simulink model "A1_acc_R2017b"  (R2017b)
settings: Solver=ode45  StartTime=0.0  StopTime=80.0  MaxStep=0.001  RelTol=1e-3
values from neighbouring files (symbols this model uses):
  a = data(2)    [A1_10.m]    (also in problem6.m = 270)
  b = data(3)    [A1_10.m]    (also in problem6.m = 11000)
  Ki = 0.0    (= 0)    [A1_10.m]
  Kp = 0.0    (= 0)    [A1_10.m]
  m = data(1)    [A1_10.m]    (also in problem6.m = 1740)
undefined symbols (not defined in the file or in its folder): Kd
settings Model: Creator=jofr  LastModifiedBy=jofr
settings DataIOCC: LimitDataPoints=on  SaveFormat=Array  SignalLoggingSaveFormat=ModelDataLogs
settings OptimizationCC: BlockReduction=off  BooleanDataType=off  LifeSpan=inf
settings DebuggingCC: SaveWithParameterizedLinksMsg=none  UnderspecifiedInitializationDetection=Classic  MergeDetectMultiDrivingBlocksExec=none  SignalResolutionControl=TryResolveAllWithWarning  MultiTaskDSMMsg=warning  MultiTaskCondExecSysMsg=none  SFUnexpectedBacktrackingDiag=warning  SFNoUnconditionalDefaultTransitionDiag=warning  SFExecutionAtInitializationDiag=none
settings HardwareCC: ProdBitPerPointer=32  ProdBitPerSizeT=32  ProdBitPerPtrDiffT=32  ProdLargestAtomicFloat=None  ProdIntDivRoundTo=Undefined  ProdEndianess=Unspecified  ProdWordSize=32  ProdHWDeviceType=32-bit Generic  TargetUnknown=on
settings ModelReferenceCC: PropagateSignalLabelsOutOfModel=off
settings CodeAppCC: StateflowObjectComments=on
settings GRTTargetCC: TargetLangStandard=C89/C90 (ANSI)
settings ConfigComp: CovMetricSettings=dw  CovSaveCumulativeToWorkspaceVar=on  CovSaveSingleToWorkspaceVar=on  CovExternalEMLEnable=off

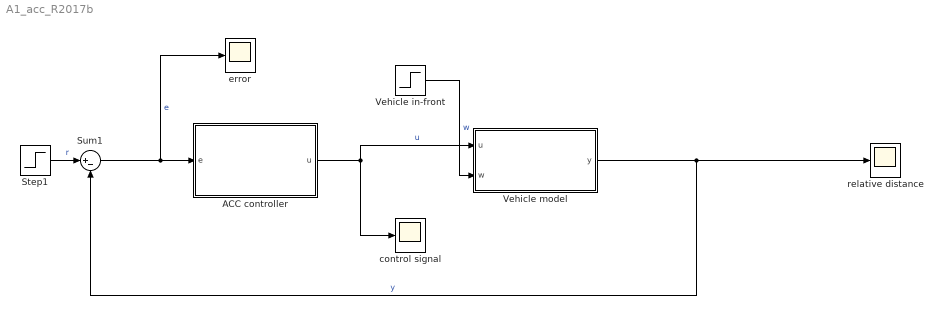
== system A1_acc_R2017b ==
  ACC controller : Subsystem
  Step1 : Step  Time=10  Before=30  After=30  SampleTime=0
  Sum1 : Sum  Inputs=|+-
  Vehicle in-front : Step  Time=10  Before=25  After=15  SampleTime=0
  Vehicle model : Subsystem
  control signal : Scope
  error : Scope
  "relative distance " : Scope
  wires:
  Sum1/1 -> ACC controller/1(e), error/1  "e"
  Step1/1 -> Sum1/1  "r"
  ACC controller/1(u) -> control signal/1, Vehicle model/1(u)  "u"
  Vehicle model/1(y) -> "relative distance "/1, Sum1/2  "y"
  Vehicle in-front/1 -> Vehicle model/2(w)  "w"

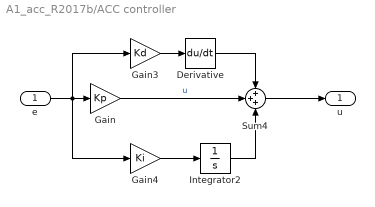
== system A1_acc_R2017b/ACC controller ==
  e : Inport
  Derivative : Derivative
  Gain : Gain  Gain=Kp
  Gain3 : Gain  Gain=Kd
  Gain4 : Gain  Gain=Ki
  Integrator2 : Integrator  InitialCondition=a*25/b
  Sum4 : Sum  Inputs=+++
  u : Outport
  wires:
  Integrator2/1 -> Sum4/3
  Sum4/1 -> u/1
  Derivative/1 -> Sum4/1
  e/1 -> Gain4/1, Gain3/1, Gain/1
  Gain/1 -> Sum4/2  "u"
  Gain4/1 -> Integrator2/1
  Gain3/1 -> Derivative/1

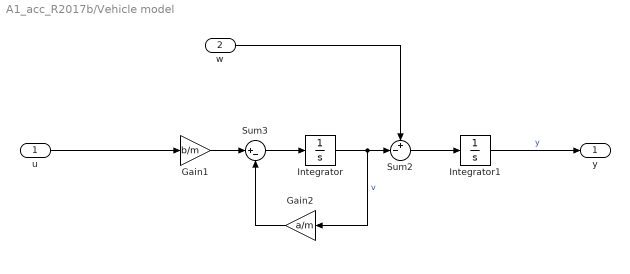
== system A1_acc_R2017b/Vehicle model ==
  u : Inport
  w : Inport  Port=2
  Gain1 : Gain  Gain=b/m
  Gain2 : Gain  Gain=a/m
  Integrator : Integrator  InitialCondition=25
  Integrator1 : Integrator  InitialCondition=30
  Sum2 : Sum  Inputs=+-|
  Sum3 : Sum  Inputs=|+-
  y : Outport
  wires:
  w/1 -> Sum2/1
  u/1 -> Gain1/1
  Integrator1/1 -> y/1  "y"
  Integrator/1 -> Sum2/2, Gain2/1  "v"
  Gain2/1 -> Sum3/2
  Sum3/1 -> Integrator/1
  Sum2/1 -> Integrator1/1
  Gain1/1 -> Sum3/1
